simulink model "Inc_1"  (R2018a)
settings: Solver=VariableStepAuto  StartTime=0.0  StopTime=10.0  RelTol=1e-3
settings Model: Creator=midog  LastModifiedBy=midog

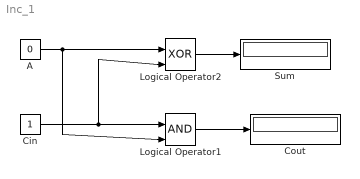
== system Inc_1 ==
  A : Constant  Value=0
  Cin : Constant
  Cout : Display
  Logical Operator1 : Logic  IconShape=distinctive  AllPortsSameDT=off  OutDataTypeStr=boolean
  Logical Operator2 : Logic  Operator=XOR  IconShape=distinctive  AllPortsSameDT=off  OutDataTypeStr=boolean
  Sum : Display
  wires:
  Logical Operator2/1 -> Sum/1
  Logical Operator1/1 -> Cout/1
  A/1 -> Logical Operator1/2, Logical Operator2/1
  Cin/1 -> Logical Operator2/2, Logical Operator1/1
